simulink model "sim_dinamica"  (R2020a)
settings: Solver=VariableStepAuto  StartTime=0.0  StopTime=25  RelTol=1e-3
undefined symbols (not defined in the file): theta_initial, torque_final, torque_initial, torque_step_time
(part 1 of 3)
settings Model: Creator=lunet  LastModifiedBy=lunet
settings DataIOCC: ReturnWorkspaceOutputs=off

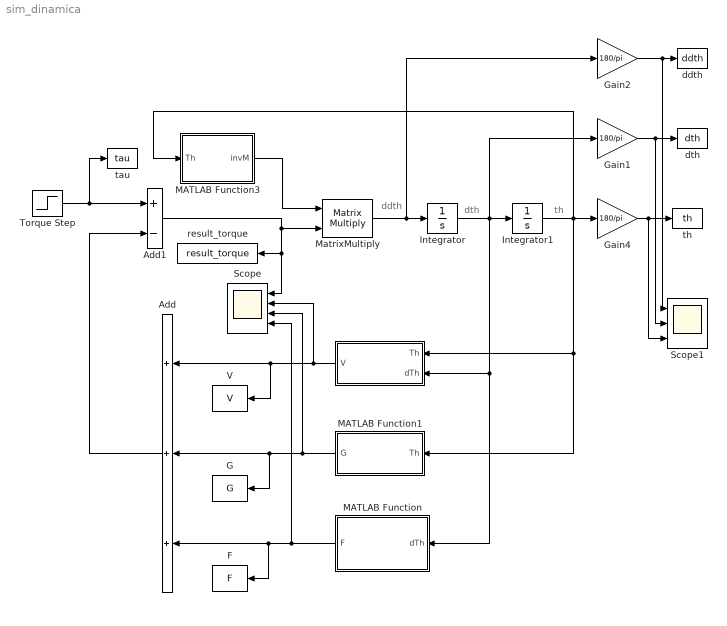
== system sim_dinamica ==
  note: ddth
  note: th
  note: dth
  " " : MATLAB Function  TreatAsAtomicUnit=on
  Add : Sum  Inputs=+++
  Add1 : Sum  Inputs=+-
  F : ToWorkspace  VariableName=F  SampleTime=-1
  G : ToWorkspace  VariableName=G  SampleTime=-1
  Gain1 : Gain  Gain=180/pi
  Gain2 : Gain  Gain=180/pi
  Gain4 : Gain  Gain=180/pi
  Integrator : Integrator  InitialCondition=[0 0 0 0 0]
  Integrator1 : Integrator  InitialCondition=theta_initial
  MATLAB Function : MATLAB Function  TreatAsAtomicUnit=on
  MATLAB Function1 : MATLAB Function  TreatAsAtomicUnit=on
  MATLAB Function3 : MATLAB Function  TreatAsAtomicUnit=on
  MatrixMultiply : Product  Multiplication=Matrix(*)
  Scope : Scope  NumInputPorts=4
  Scope1 : Scope  NumInputPorts=3
  Torque Step : Step  Time=torque_step_time  Before=torque_initial  After=torque_final  SampleTime=0
  V : ToWorkspace  VariableName=V  SampleTime=-1
  ddth : ToWorkspace  VariableName=ddth  SampleTime=-1
  dth : ToWorkspace  VariableName=dth  SampleTime=-1
  result_torque : ToWorkspace  VariableName=result_torque  SampleTime=-1
  tau : ToWorkspace  VariableName=tau  SampleTime=-1
  th : ToWorkspace  VariableName=th  SampleTime=-1
  wires:
  MATLAB Function3/1(invM) -> MatrixMultiply/1
  MatrixMultiply/1 -> Integrator/1, Gain2/1
  Integrator/1 -> Integrator1/1, Gain1/1, " "/2(dTh), MATLAB Function/1(dTh)
  Integrator1/1 -> " "/1(Th), MATLAB Function1/1(Th), MATLAB Function3/1(Th), Gain4/1
  " "/1(V) -> Scope/2, Add/1, V/1
  MATLAB Function1/1(G) -> Scope/3, G/1, Add/2
  MATLAB Function/1(F) -> Scope/4, F/1, Add/3
  Add1/1 -> result_torque/1, Scope/1, MatrixMultiply/2
  Add/1 -> Add1/2
  Gain4/1 -> Scope1/3, th/1
  Gain1/1 -> Scope1/2, dth/1
  Gain2/1 -> Scope1/1, ddth/1
  Torque Step/1 -> tau/1, Add1/1

== matlab function sim_dinamica/MATLAB Function1 ==
  data: Th input; G output
function G = calcul_G(Th)

th1 = Th(1);
th2 = Th(2);
th3 = Th(3);
th4 = Th(4);
th5 = Th(5);
g = 9.81;

G = [                                                                                                                                                                                                                                                                                               0;
 -g*((49*cos(th2)*sin(th3))/125 - cos(th2)/2 + (49*cos(th3)*sin(th2))/125 + (3*cos(th2)*cos(th5)*sin(th3))/40 + (3*cos(th3)*cos(th5)*sin(th2))/40 + (3*cos(th2)*cos(th3)*cos(th4)*sin(th5))/40 - (3*cos(th4)*sin(th2)*sin(th3)*sin(th5))/40);
                 -g*((49*cos(th2)*sin(th3))/125 + (49*cos(th3)*sin(th2))/125 + (3*cos(th2)*cos(th5)*sin(th3))/40 + (3*cos(th3)*cos(th5)*sin(th2))/40 + (3*cos(th2)*cos(th3)*cos(th4)*sin(th5))/40 - (3*cos(th4)*sin(th2)*sin(th3)*sin(th5))/40);
                                                                                                                                                                                                                                                (3*g*sin(th4)*sin(th5)*sin(th2 + th3))/40;
                                                                                       -g*((3*cos(th2)*cos(th3)*sin(th5))/40 - (3*sin(th2)*sin(th3)*sin(th5))/40 + (3*cos(th2)*cos(th4)*cos(th5)*sin(th3))/40 + (3*cos(th3)*cos(th4)*cos(th5)*sin(th2))/40)];

== matlab function sim_dinamica/MATLAB Function3 ==
  data: Th input; invM output
function invM = calcul_invM(Th)

th1 = Th(1);
th2 = Th(2);
th3 = Th(3);
th4 = Th(4);
th5 = Th(5);

M = [ (87*cos(th2)^2*cos(th5))/2500 + (87*cos(th3)^2*cos(th5))/2500 - (33*cos(th2)^2*sin(th3))/50 + (53231*cos(th2)^2)/62500 + (8453*cos(th3)^2)/31250 - (9*cos(th5)^2)/3200 - (8453*cos(th2)^2*cos(th3)^2)/15625 - (217*cos(th2)^2*cos(th4)^2)/80000 + (9*cos(th2)^2*cos(th5)^2)/3200 - (217*cos(th3)^2*cos(th4)^2)/80000 + (9*cos(th3)^2*cos(th5)^2)/3200 - (87*cos(th2)^2*cos(th3)^2*cos(th5))/1250 - (33*cos(th2)*cos(th3)*sin(th2))/50 + (217*cos(th2)^2*cos(th3)^2*cos(th4)^2)/40000 - (9*cos(th2)^2*cos(th3)^2*cos(th5)^2)/1600 + (9*cos(th2)^2*cos(th4)^2*cos(th5)^2)/3200 + (9*cos(th3)^2*cos(th4)^2*cos(th5)^2)/3200 - (3*cos(th2)^2*cos(th5)*sin(th3))/80 - (9*cos(th2)^2*cos(th3)^2*cos(th4)^2*cos(th5)^2)/1600 - (3*cos(th2)*cos(th3)*cos(th5)*sin(th2))/80 + (8453*cos(th2)*cos(th3)*sin(th2)*sin(th3))/15625 - (87*cos(th2)*cos(th4)*sin(th2)*sin(th5))/2500 - (87*cos(th3)*cos(th4)*sin(th3)*sin(th5))/2500 - (3*cos(th2)^2*cos(th3)*cos(th4)*sin(th5))/80 + (3*cos(th2)*cos(th4)*sin(th2)*sin(th3)*sin(th5))/80 - (217*cos(th2)*cos(th3)*cos(th4)^2*sin(th2)*sin(th3))/40000 + (9*cos(th2)*cos(th3)*cos(th5)^2*sin(th2)*sin(th3))/1600 + (87*cos(th2)*cos(th3)^2*cos(th4)*sin(th2)*sin(th5))/1250 + (87*cos(th2)^2*cos(th3)*cos(th4)*sin(th3)*sin(th5))/1250 + (87*cos(th2)*cos(th3)*cos(th5)*sin(th2)*sin(th3))/1250 - (9*cos(th2)*cos(th4)*cos(th5)*sin(th2)*sin(th5))/1600 - (9*cos(th3)*cos(th4)*cos(th5)*sin(th3)*sin(th5))/1600 + (9*cos(th2)*cos(th3)*cos(th4)^2*cos(th5)^2*sin(th2)*sin(th3))/1600 + (9*cos(th2)*cos(th3)^2*cos(th4)*cos(th5)*sin(th2)*sin(th5))/800 + (9*cos(th2)^2*cos(th3)*cos(th4)*cos(th5)*sin(th3)*sin(th5))/800 + 3793/80000, -(sin(th4)*(1500*sin(th2)*sin(th5) - 217*cos(th2)*cos(th4)*sin(th3) - 217*cos(th3)*cos(th4)*sin(th2) + 1392*cos(th2)*cos(th3)*sin(th5) - 1392*sin(th2)*sin(th3)*sin(th5) + 225*cos(th2)*cos(th3)*cos(th5)*sin(th5) - 225*cos(th5)*sin(th2)*sin(th3)*sin(th5) + 225*cos(th2)*cos(th4)*cos(th5)^2*sin(th3) + 225*cos(th3)*cos(th4)*cos(th5)^2*sin(th2)))/80000, (sin(th4)*(217*cos(th2)*cos(th4)*sin(th3) + 217*cos(th3)*cos(th4)*sin(th2) - 1392*cos(th2)*cos(th3)*sin(th5) + 1392*sin(th2)*sin(th3)*sin(th5) - 225*cos(th2)*cos(th3)*cos(th5)*sin(th5) + 225*cos(th5)*sin(th2)*sin(th3)*sin(th5) - 225*cos(th2)*cos(th4)*cos(th5)^2*sin(th3) - 225*cos(th3)*cos(th4)*cos(th5)^2*sin(th2)))/80000, (489*cos(th2)*cos(th3))/80000 - (489*sin(th2)*sin(th3))/80000 - (3*cos(th2)*cos(th4)*sin(th5))/160 - (9*cos(th2)*cos(th3)*cos(th5)^2)/3200 + (9*cos(th5)^2*sin(th2)*sin(th3))/3200 + (87*cos(th2)*cos(th4)*sin(th3)*sin(th5))/5000 + (87*cos(th3)*cos(th4)*sin(th2)*sin(th5))/5000 + (9*cos(th2)*cos(th4)*cos(th5)*sin(th3)*sin(th5))/3200 + (9*cos(th3)*cos(th4)*cos(th5)*sin(th2)*sin(th5))/3200, (sin(th4)*(353*cos(th2)*sin(th3) + 353*cos(th3)*sin(th2) - 1500*cos(th2)*cos(th5) + 1392*cos(th2)*cos(th5)*sin(th3) + 1392*cos(th3)*cos(th5)*sin(th2)))/80000;
                                                                                                                                                                                                                                                                                                                                                                                                                                                                                                                                                                                                                                                                                                                                                                                                                                                                                                                                                                                                                                                                                                                                                                                                                                                                                                                                                                                                                                                                                                                                                                                            -(sin(th4)*(1500*sin(th2)*sin(th5) - 217*cos(th2)*cos(th4)*sin(th3) - 217*cos(th3)*cos(th4)*sin(th2) + 1392*cos(th2)*cos(th3)*sin(th5) - 1392*sin(th2)*sin(th3)*sin(th5) + 225*cos(th2)*cos(th3)*cos(th5)*sin(th5) - 225*cos(th5)*sin(th2)*sin(th3)*sin(th5) + 225*cos(th2)*cos(th4)*cos(th5)^2*sin(th3) + 225*cos(th3)*cos(th4)*cos(th5)^2*sin(th2)))/80000,                                                                                                                                                                                                                       (87*cos(th5))/2500 - (33*sin(th3))/50 - (3*cos(th5)*sin(th3))/80 + (217*cos(th4)^2)/80000 + (9*cos(th5)^2)/3200 - (9*cos(th4)^2*cos(th5)^2)/3200 - (3*cos(th3)*cos(th4)*sin(th5))/80 + 54781/62500,                                                                                                                                                                                   (87*cos(th5))/2500 - (33*sin(th3))/100 - (3*cos(th5)*sin(th3))/160 + (217*cos(th4)^2)/80000 + (9*cos(th5)^2)/3200 - (9*cos(th4)^2*cos(th5)^2)/3200 - (3*cos(th3)*cos(th4)*sin(th5))/160 + 72749/250000,                                                                                                                                                                                                                                                                                                                                                                                                                     -(3*sin(th4)*sin(th5)*(75*cos(th5) - 500*sin(th3) + 464))/80000,                                                          (353*cos(th4))/80000 - (3*cos(th3)*sin(th5))/160 + (87*cos(th4)*cos(th5))/5000 - (3*cos(th4)*cos(th5)*sin(th3))/160;
                                                                                                                                                                                                                                                                                                                                                                                                                                                                                                                                                                                                                                                                                                                                                                                                                                                                                                                                                                                                                                                                                                                                                                                                                                                                                                                                                                                                                                                                                                                                                                                                                            (sin(th4)*(217*cos(th2)*cos(th4)*sin(th3) + 217*cos(th3)*cos(th4)*sin(th2) - 1392*cos(th2)*cos(th3)*sin(th5) + 1392*sin(th2)*sin(th3)*sin(th5) - 225*cos(th2)*cos(th3)*cos(th5)*sin(th5) + 225*cos(th5)*sin(th2)*sin(th3)*sin(th5) - 225*cos(th2)*cos(th4)*cos(th5)^2*sin(th3) - 225*cos(th3)*cos(th4)*cos(th5)^2*sin(th2)))/80000,                                                                                                                                                                                                                   (87*cos(th5))/2500 - (33*sin(th3))/100 - (3*cos(th5)*sin(th3))/160 + (217*cos(th4)^2)/80000 + (9*cos(th5)^2)/3200 - (9*cos(th4)^2*cos(th5)^2)/3200 - (3*cos(th3)*cos(th4)*sin(th5))/160 + 72749/250000,                                                                                                                                                                                                                                                                                          (87*cos(th5))/2500 + (217*cos(th4)^2)/80000 + (9*cos(th5)^2)/3200 - (9*cos(th4)^2*cos(th5)^2)/3200 + 72749/250000,                                                                                                                                                                                                                                                                                                                                                                                                                                       -(3*sin(th4)*sin(th5)*(75*cos(th5) + 464))/80000,                                                                                                                                                         (cos(th4)*(1392*cos(th5) + 353))/80000;
                                                                                                                                                                                                                                                                                                                                                                                                                                                                                                                                                                                                                                                                                                                                                                                                                                                                                                                                                                                                                                                                                                                                                                                                                                                                                                                                                                                                                                                                                                                                                      (489*cos(th2)*cos(th3))/80000 - (489*sin(th2)*sin(th3))/80000 - (3*cos(th2)*cos(th4)*sin(th5))/160 - (9*cos(th2)*cos(th3)*cos(th5)^2)/3200 + (9*cos(th5)^2*sin(th2)*sin(th3))/3200 + (87*cos(th2)*cos(th4)*sin(th3)*sin(th5))/5000 + (87*cos(th3)*cos(th4)*sin(th2)*sin(th5))/5000 + (9*cos(th2)*cos(th4)*cos(th5)*sin(th3)*sin(th5))/3200 + (9*cos(th3)*cos(th4)*cos(th5)*sin(th2)*sin(th5))/3200,                                                                                                                                                                                                                                                                                                                                                                               -(3*sin(th4)*sin(th5)*(75*cos(th5) - 500*sin(th3) + 464))/80000,                                                                                                                                                                                                                                                                                                                                                                 -(3*sin(th4)*sin(th5)*(75*cos(th5) + 464))/80000,                                                                                                                                                                                                                                                                                                                                                                                                                                                              489/80000 - (9*cos(th5)^2)/3200,                                                                                                                                                                                                    0;
                                                                                                                                                                                                                                                                                                                                                                                                                                                                                                                                                                                                                                                                                                                                                                                                                                                                                                                                                                                                                                                                                                                                                                                                                                                                                                                                                                                                                                                                                                                                                                                                                                                                                                                                                                                                                                                 (sin(th4)*(353*cos(th2)*sin(th3) + 353*cos(th3)*sin(th2) - 1500*cos(th2)*cos(th5) + 1392*cos(th2)*cos(th5)*sin(th3) + 1392*cos(th3)*cos(th5)*sin(th2)))/80000,                                                                                                                                                                                                                                                                                                               (353*cos(th4))/80000 - (3*cos(th3)*sin(th5))/160 + (87*cos(th4)*cos(th5))/5000 - (3*cos(th4)*cos(th5)*sin(th3))/160,                                                                                                                                                                                                                                                                                                                                                                              (cos(th4)*(1392*cos(th5) + 353))/80000,                                                                                                                                                                                                                                                                                                                                                                                                                                                                                               0,                                                                                                                                                                                            353/80000];
                                                                                                                                                                                                                                                                                                                                                                                                                                                                                                                                                                                                                                                                                                                                                                                                                                                                                                                                                                                                                                                                                                                                                                                                                                                                                                                                                                                                                                                                                                                                                                                                                                                                                                                                                                                                                                             
invM = M^-1;
